simulink model "Seesaw_Full"  (R2024b)
settings: Solver=ode45  StartTime=0.0  StopTime=10  MaxStep=1e-3  RelTol=1e-4  AbsTol=1e-6
undefined symbols (not defined in the file): A_input, f_input
settings Model: Creator=Karim Negm  LastModifiedBy=Karim Negm

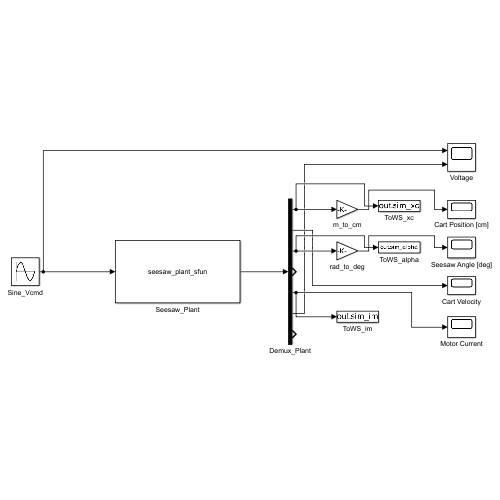
[thumbnail: Simulink's stored preview of the top-level diagram]
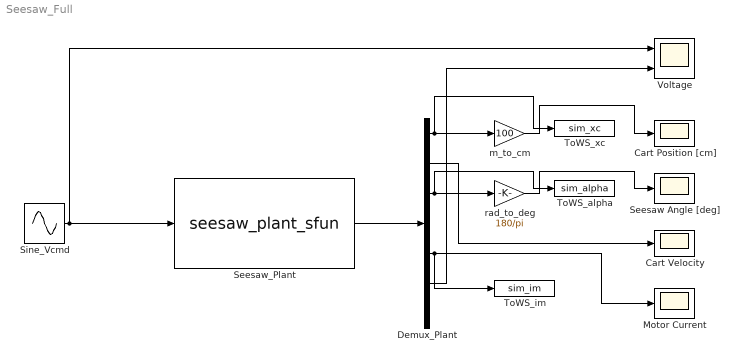
== system Seesaw_Full ==
  Cart Position [cm] : Scope
  Cart Velocity : Scope
  Demux_Plant : Demux  Outputs=7
  Motor Current : Scope
  Seesaw Angle [deg] : Scope
  Seesaw_Plant : M-S-Function  FunctionName=seesaw_plant_sfun
  Sine_Vcmd : Sin  Amplitude=A_input  Frequency=2*pi*f_input  SampleTime=0
  ToWS_alpha : ToWorkspace  VariableName=sim_alpha  SaveFormat=Timeseries  SampleTime=-1
  ToWS_im : ToWorkspace  VariableName=sim_im  SaveFormat=Timeseries  SampleTime=-1
  ToWS_xc : ToWorkspace  VariableName=sim_xc  SaveFormat=Timeseries  SampleTime=-1
  Voltage : Scope  NumInputPorts=2
  m_to_cm : Gain  Gain=100
  rad_to_deg : Gain  Gain=180/pi
  wires:
  Sine_Vcmd/1 -> Seesaw_Plant/1, Voltage/1
  Seesaw_Plant/1 -> Demux_Plant/1
  Demux_Plant/1 -> m_to_cm/1, ToWS_xc/1
  m_to_cm/1 -> Cart Position [cm]/1
  Demux_Plant/2 -> Cart Velocity/1
  Demux_Plant/3 -> rad_to_deg/1, ToWS_alpha/1
  rad_to_deg/1 -> Seesaw Angle [deg]/1
  Demux_Plant/5 -> Motor Current/1, ToWS_im/1
  Demux_Plant/6 -> Voltage/2
